simulink model "ExampleVehicleSpeed"  (R2021a)
settings: Solver=VariableStepAuto  StartTime=0.0  StopTime=10.0  RelTol=1e-3
settings Model: Creator=Tyler  LastModifiedBy=Tyler

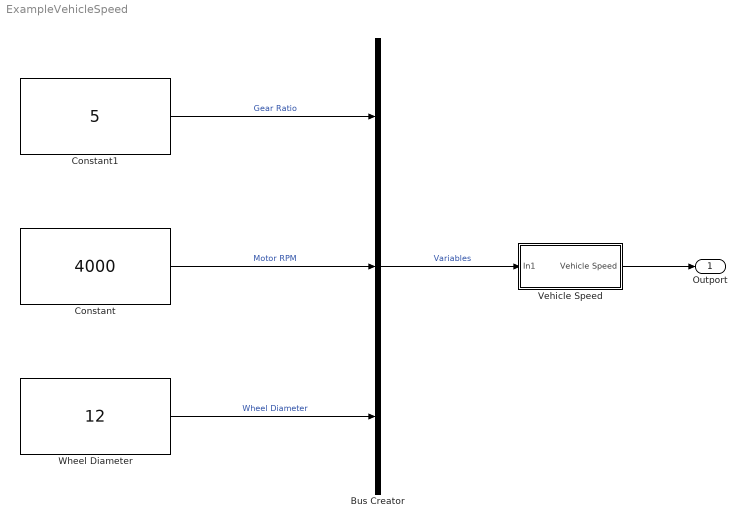
== system ExampleVehicleSpeed ==
  Bus Creator : BusCreator  Inputs=3
  Constant : Constant  Value=4000
  Constant1 : Constant  Value=5
  Vehicle Speed : Subsystem
  Wheel Diameter : Constant  Value=12
  Outport : Outport
  wires:
  Constant1/1 -> Bus Creator/1  "Gear Ratio"
  Constant/1 -> Bus Creator/2  "Motor RPM"
  Bus Creator/1 -> Vehicle Speed/1(In1)  "Variables"
  Wheel Diameter/1 -> Bus Creator/3  "Wheel Diameter"
  Vehicle Speed/1(Vehicle Speed) -> Outport/1

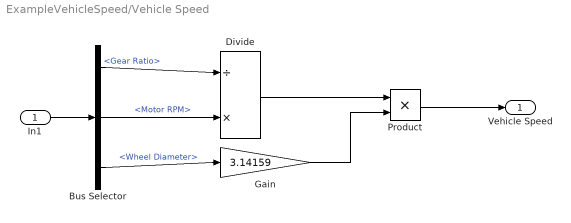
== system ExampleVehicleSpeed/Vehicle Speed ==
  In1 : Inport
  Bus Selector : BusSelector  OutputSignals=Gear Ratio,Motor RPM,Wheel Diameter
  Divide : Product  Inputs=/*
  Gain : Gain  Gain=3.14159
  Product : Product
  Vehicle Speed : Outport
  wires:
  In1/1 -> Bus Selector/1
  Bus Selector/1 -> Divide/1  "<Gear Ratio>"
  Bus Selector/2 -> Divide/2  "<Motor RPM>"
  Bus Selector/3 -> Gain/1  "<Wheel Diameter>"
  Divide/1 -> Product/1
  Gain/1 -> Product/2
  Product/1 -> Vehicle Speed/1
